simulink model "dosing_sgs"  (R2018a)
settings: Solver=FixedStepDiscrete  StartTime=0.0  StopTime=500  FixedStep=1  RelTol=1e-3
settings Model: Creator=Home  LastModifiedBy=Home

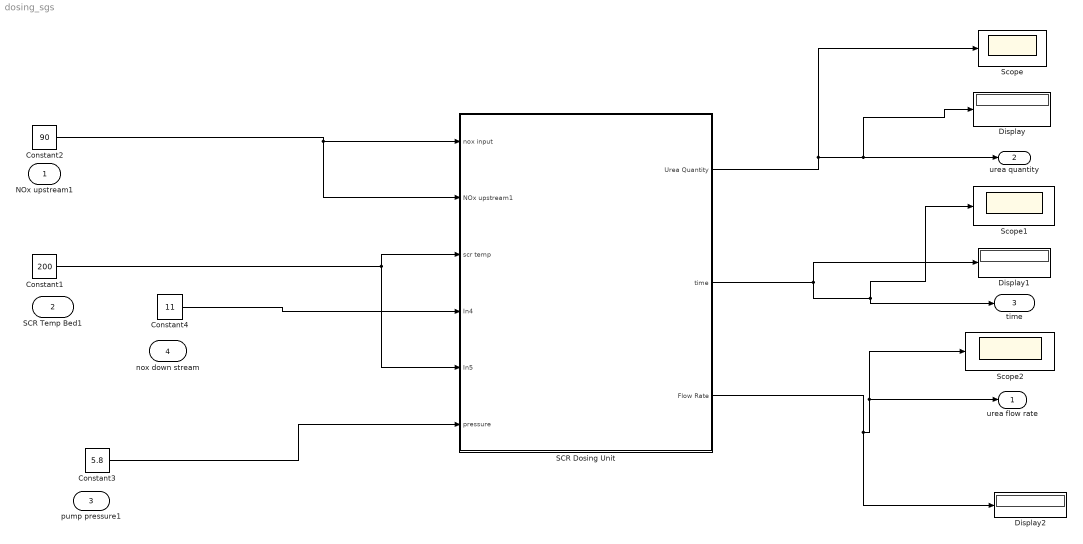
== system dosing_sgs ==
  NOx upstream1 : Inport
  SCR Temp Bed1 : Inport  Port=2
  pump pressure1 : Inport  Port=3
  nox down stream : Inport  Port=4
  Constant1 : Constant  Value=200
  Constant2 : Constant  Value=90
  Constant3 : Constant  Value=5.8
  Constant4 : Constant  Value=11
  Display : Display
  Display1 : Display
  Display2 : Display
  SCR Dosing Unit : Subsystem
  Scope : Scope
  Scope1 : Scope
  Scope2 : Scope
  urea flow rate : Outport
  urea quantity : Outport  Port=2
  "time " : Outport  Port=3
  wires:
  Constant3/1 -> SCR Dosing Unit/6(pressure)
  SCR Dosing Unit/1(Urea Quantity) -> Scope/1, Display/1, urea quantity/1
  SCR Dosing Unit/2("time ") -> Display1/1, Scope1/1, "time "/1
  SCR Dosing Unit/3(Flow Rate) -> Display2/1, Scope2/1, urea flow rate/1
  Constant2/1 -> SCR Dosing Unit/2(NOx upstream1), SCR Dosing Unit/1(nox input)
  Constant1/1 -> SCR Dosing Unit/5(In5), SCR Dosing Unit/3(scr temp)
  Constant4/1 -> SCR Dosing Unit/4(In4)

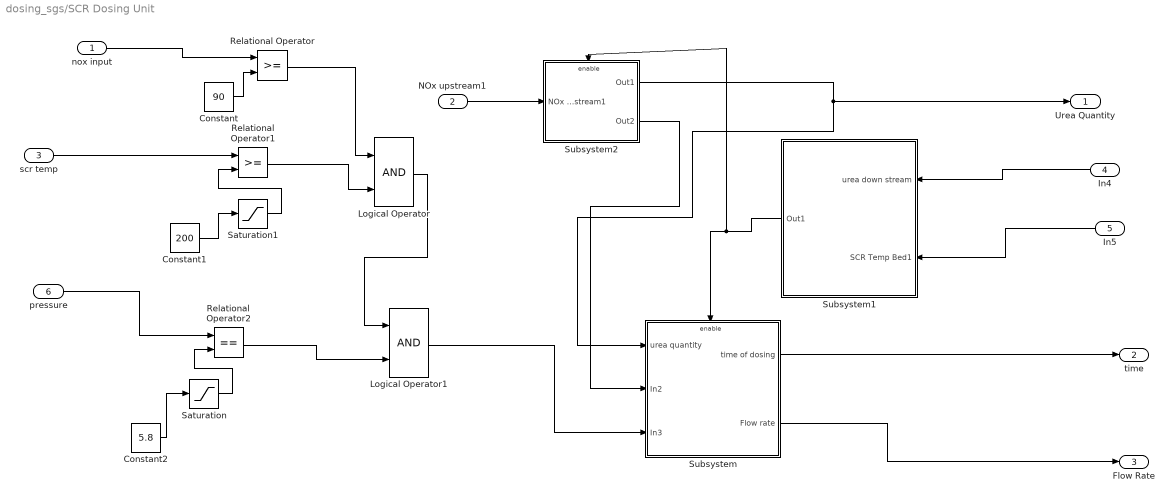
== system dosing_sgs/SCR Dosing Unit ==
  nox input : Inport
  NOx upstream1 : Inport  Port=2
  scr temp : Inport  Port=3
  In4 : Inport  Port=4
  In5 : Inport  Port=5
  pressure : Inport  Port=6
  Constant : Constant  Value=90
  Constant1 : Constant  Value=200
  Constant2 : Constant  Value=5.8
  Logical Operator : Logic  AllPortsSameDT=off  OutDataTypeStr=boolean
  Logical Operator1 : Logic  AllPortsSameDT=off  OutDataTypeStr=boolean
  Relational Operator : RelationalOperator  OutDataTypeStr=boolean  RndMeth=Simplest
  Relational Operator1 : RelationalOperator  OutDataTypeStr=boolean  RndMeth=Simplest
  Relational Operator2 : RelationalOperator  Operator===  OutDataTypeStr=boolean  RndMeth=Simplest
  Saturation : Saturate  UpperLimit=6.5  LowerLimit=5.5
  Saturation1 : Saturate  UpperLimit=700  LowerLimit=100
  Subsystem : Subsystem
  Subsystem1 : Subsystem
  Subsystem2 : Subsystem
  Urea Quantity : Outport
  "time " : Outport  Port=2
  Flow Rate : Outport  Port=3
  wires:
  Relational Operator2/1 -> Logical Operator1/2
  Constant2/1 -> Saturation/1
  Saturation/1 -> Relational Operator2/2
  Saturation1/1 -> Relational Operator1/2
  Subsystem/2(Flow rate) -> Flow Rate/1
  In4/1 -> Subsystem1/1(urea down stream)
  Constant/1 -> Relational Operator/2
  Logical Operator/1 -> Logical Operator1/1
  Relational Operator/1 -> Logical Operator/1
  Subsystem1/1(Out1) -> Subsystem2/Enable, Subsystem/Enable
  Logical Operator1/1 -> Subsystem/3(In3)
  In5/1 -> Subsystem1/2(SCR Temp Bed1)
  Constant1/1 -> Saturation1/1
  Relational Operator1/1 -> Logical Operator/2
  nox input/1 -> Relational Operator/1
  pressure/1 -> Relational Operator2/1
  Subsystem/1(time of dosing) -> "time "/1
  scr temp/1 -> Relational Operator1/1
  Subsystem2/1(Out1) -> Subsystem/1(urea quantity), Urea Quantity/1
  NOx upstream1/1 -> Subsystem2/1(NOx upstream1)
  Subsystem2/2(Out2) -> Subsystem/2(In2)

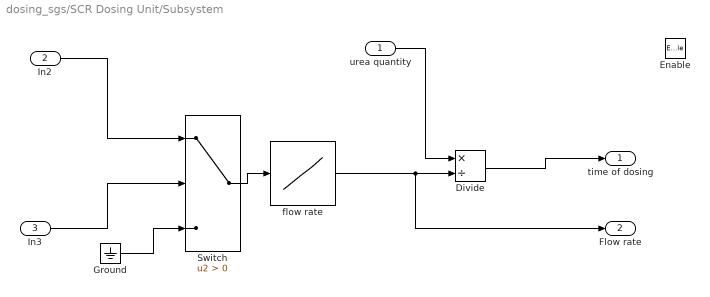
== system dosing_sgs/SCR Dosing Unit/Subsystem ==
  urea quantity : Inport
  In2 : Inport  Port=2
  In3 : Inport  Port=3
  Enable : EnablePort
  Divide : Product  Inputs=*/
  Ground : Ground
  Switch : Switch  Criteria=u2 > Threshold
  flow rate : Lookup_n-D  NumberOfTableDimensions=1  BreakpointsForDimension1=|  Table=|  InternalRulePriority=Speed  RndMeth=Simplest  InputSameDT=on
      BreakpointsForDimension1=|
      | [90
      | 96
      | 101
      | 106
      | 112
      | 117
      | 123
      | 128
      | 134
      | 139
      | 145
      | 150
      | 173
      | 197
      | 220
      | 243.3
      | 266.7
      | 290
      | 313.3
      | 336.7
      | 360
      | 383
      | 406.7
      | 438
      | 453
      | 476.7
      | 500]
      Table=|
      | [4
      | 5
      | 6
      | 7
      | 8
      | 9
      | 10
      | 11
      | 12
      | 13
      | 14
      | 15
      | 16
      | 17
      | 18
      | 19
      | 20
      | 21
      | 22
      | 23
      | 24
      | 25
      | 26
      | 27
      | 28
      | 29
      | 30]
  time of dosing : Outport
  Flow rate : Outport  Port=2
  wires:
  Ground/1 -> Switch/3
  Switch/1 -> flow rate/1
  flow rate/1 -> Flow rate/1, Divide/2
  urea quantity/1 -> Divide/1
  Divide/1 -> time of dosing/1
  In2/1 -> Switch/1
  In3/1 -> Switch/2

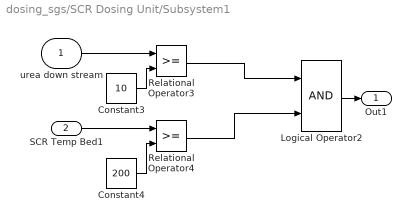
== system dosing_sgs/SCR Dosing Unit/Subsystem1 ==
  urea down stream : Inport
  SCR Temp Bed1 : Inport  Port=2
  Constant3 : Constant  Value=10
  Constant4 : Constant  Value=200
  Logical Operator2 : Logic  AllPortsSameDT=off  OutDataTypeStr=boolean
  Relational Operator3 : RelationalOperator  OutDataTypeStr=boolean  RndMeth=Simplest
  Relational Operator4 : RelationalOperator  OutDataTypeStr=boolean  RndMeth=Simplest
  Out1 : Outport
  wires:
  Relational Operator4/1 -> Logical Operator2/2
  Relational Operator3/1 -> Logical Operator2/1
  urea down stream/1 -> Relational Operator3/1
  Constant4/1 -> Relational Operator4/2
  SCR Temp Bed1/1 -> Relational Operator4/1
  Constant3/1 -> Relational Operator3/2
  Logical Operator2/1 -> Out1/1

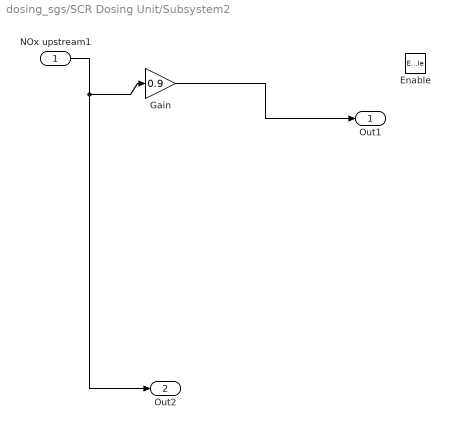
== system dosing_sgs/SCR Dosing Unit/Subsystem2 ==
  NOx upstream1 : Inport
  Enable : EnablePort
  Gain : Gain  Gain=0.9
  Out1 : Outport
  Out2 : Outport  Port=2
  wires:
  NOx upstream1/1 -> Out2/1, Gain/1
  Gain/1 -> Out1/1
